simulink model "SMA_spring_pid"  (R2018a)
settings: Solver=ode15s  StartTime=0.0  StopTime=3.5  RelTol=1e-9  AbsTol=1e-9  EnableMultiTasking=on
values from neighbouring files (symbols this model uses):
  task_params = struct    [run.m]
undefined symbols (not defined in the file or in its folder): params_BIAS
settings Model: Creator=Gianluca  LastModifiedBy=tim
settings SolverCC: AutoScaleAbsTol=off
settings DataIOCC: LimitDataPoints=on  SaveFormat=Array
settings OptimizationCC: LifeSpan=inf
settings DebuggingCC: UnderspecifiedInitializationDetection=Classic  MergeDetectMultiDrivingBlocksExec=none  SolverPrmCheckMsg=warning  StateNameClashWarn=warning  SFUnexpectedBacktrackingDiag=warning  SFNoUnconditionalDefaultTransitionDiag=warning  SFExecutionAtInitializationDiag=none
settings HardwareCC: ProdBitPerPointer=32  ProdBitPerSizeT=32  ProdBitPerPtrDiffT=32  ProdLargestAtomicFloat=None  ProdIntDivRoundTo=Undefined  ProdEndianess=Unspecified  ProdWordSize=32  ProdHWDeviceType=32-bit Generic
settings ModelReferenceCC: PropagateSignalLabelsOutOfModel=off
settings CodeAppCC: StateflowObjectComments=on
settings GRTTargetCC: TargetLangStandard=C89/C90 (ANSI)  GeneratePreprocessorConditionals=Disable all
settings ConfigComp: CovMetricSettings=dw  CovHtmlReporting=on  CovSaveCumulativeToWorkspaceVar=on  CovSaveSingleToWorkspaceVar=on  CovExternalEMLEnable=off

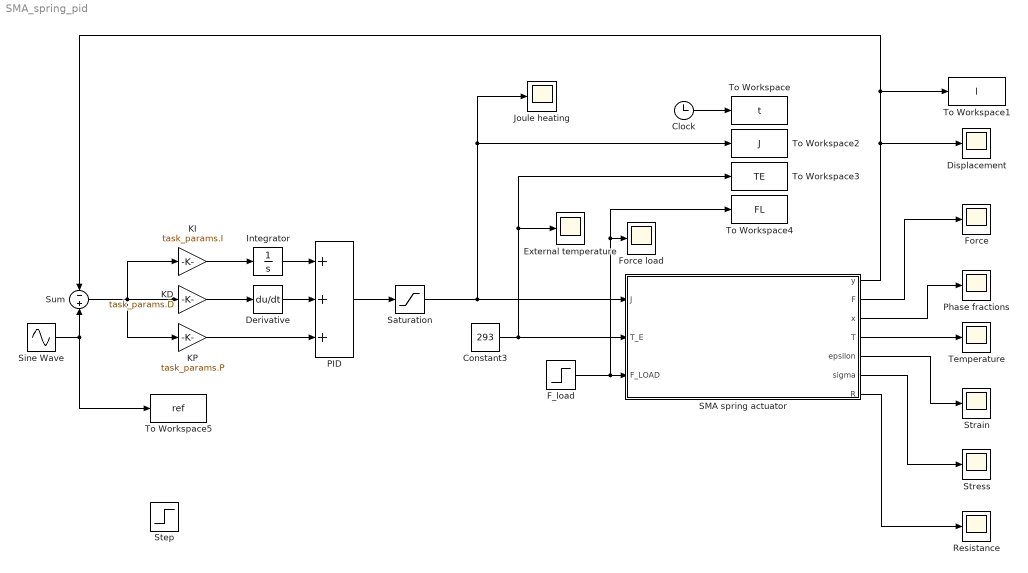
== system SMA_spring_pid ==
  " Force load" : Scope
  Clock : Clock
  Constant3 : Constant  Value=293
  Derivative : Derivative
  Displacement : Scope
  External temperature : Scope
  F_load : Step  After=0.05*0  SampleTime=0
  Force : Scope
  Integrator : Integrator
  Joule heating : Scope
  KD : Gain  Gain=task_params.D
  KI : Gain  Gain=task_params.I
  KP : Gain  Gain=task_params.P
  PID : Sum  Inputs=+++
  Phase fractions : Scope
  Resistance : Scope
  SMA spring actuator : Subsystem
      mask Display:
      | color('black');
      | patch(3*[-1 1 1 -1],1.1*[-1 -1 1 1],[1 1 1]);
      | patch([-1.6 -0.8],[-0.9 0.3],[0 0 0]);
      | patch([-0.8 1.2],[0.3 0.3],[0 0 0]);
      | patch([1.6 0.8],[0.9 -0.3],[0 0 0]);
      | patch([0.8 -1.2],[-0.3 -0.3],[0 0 0]);
      | disp('SMA spring');
      | 
      | color('blue');
      | port_label('input', 1, 'J [W]','texmode','on');
      | port_label('input', 2, 'T_E [K]','texmode','on');
      | port_label('input', 3, 'F_{LOAD} [N]','texmode','on');
      | 
      | color('red');
      | port_label('output', 1, 'y [m]','texmode','on');
      | port_label('output', 2, 'F [N]','texmode','on');
      | port_label('output', 3, 'x_+, x_-, x_A [-]','texmode','on');
      | port_label('output', 4, 'T [K]','texmode','on');
      | port_label('output', 5, '\epsilon [-]','texmode','on');
      | port_label('output', 6, '\sigma [Pa]','texmode','on');
      | port_label('output', 7, 'R [\Omega]','texmode','on');
  Saturation : Saturate  UpperLimit=0.25  LowerLimit=0  ZeroCross=off
  Sine Wave : Sin  Amplitude=task_params.sine_A  Bias=task_params.sine_bias  Frequency=2 * pi * task_params.sine_f  SampleTime=0
  Step : Step  Time=0  After=0.25*0.5  SampleTime=0
  Strain : Scope
  Stress : Scope
  Sum : Sum  Inputs=-+
  Temperature : Scope
  To Workspace : ToWorkspace  VariableName=t  SampleTime=0.01
  To Workspace1 : ToWorkspace  VariableName=l  SampleTime=0.01
  To Workspace2 : ToWorkspace  VariableName=J  SampleTime=0.01
  To Workspace3 : ToWorkspace  VariableName=TE  SampleTime=0.01
  To Workspace4 : ToWorkspace  VariableName=FL  SampleTime=0.01
  To Workspace5 : ToWorkspace  VariableName=ref  SampleTime=0.01
  wires:
  Constant3/1 -> To Workspace3/1, External temperature/1, SMA spring actuator/2(T_E)
  F_load/1 -> To Workspace4/1, " Force load"/1, SMA spring actuator/3(F_LOAD)
  SMA spring actuator/1(y) -> To Workspace1/1, Sum/1, Displacement/1
  SMA spring actuator/2(F) -> Force/1
  SMA spring actuator/3(x) -> Phase fractions/1
  SMA spring actuator/4(T) -> Temperature/1
  SMA spring actuator/5(epsilon) -> Strain/1
  SMA spring actuator/6(sigma) -> Stress/1
  SMA spring actuator/7(R) -> Resistance/1
  PID/1 -> Saturation/1
  Clock/1 -> To Workspace/1
  Saturation/1 -> Joule heating/1, To Workspace2/1, SMA spring actuator/1(J)
  Integrator/1 -> PID/1
  KP/1 -> PID/3
  Derivative/1 -> PID/2
  KI/1 -> Integrator/1
  Sum/1 -> KP/1, KI/1, KD/1
  KD/1 -> Derivative/1
  Sine Wave/1 -> To Workspace5/1, Sum/2

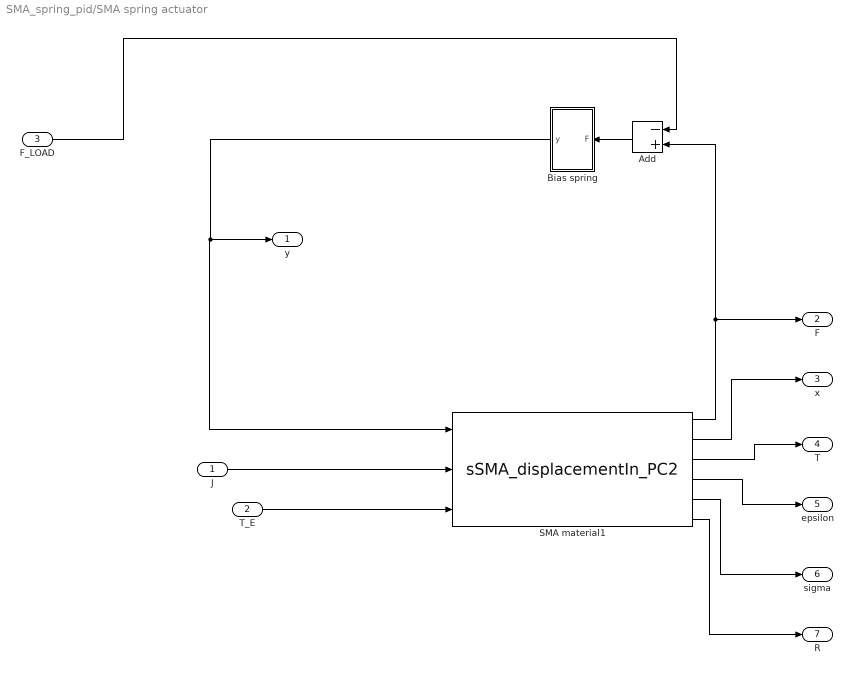
== system SMA_spring_pid/SMA spring actuator ==
  J : Inport
  T_E : Inport  Port=2
  F_LOAD : Inport  Port=3
  Add : Sum  Inputs=-+
  Bias spring : Subsystem
  SMA material1 : M-S-Function  FunctionName=sSMA_displacementIn_PC2  Parameters=params_PC2, initConds_PC2
      mask Display:
      | color('black');
      | patch(3*[-1 1 1 -1],1.1*[-1 -1 1 1],[1 1 1]);
      | patch([-1.6 -0.8],[-0.9 0.3],[0 0 0]);
      | patch([-0.8 1.2],[0.3 0.3],[0 0 0]);
      | patch([1.6 0.8],[0.9 -0.3],[0 0 0]);
      | patch([0.8 -1.2],[-0.3 -0.3],[0 0 0]);
      | disp('SMA');
      | 
      | color('blue');
      | port_label('input', 1, 'y [m]','texmode','on');
      | port_label('input', 2, 'J [W]','texmode','on');
      | port_label('input', 3, 'T_E [K]','texmode','on');
      | 
      | color('red');
      | port_label('output', 1, 'F [N]','texmode','on');
      | port_label('output', 2, 'x_+, x_-, x_A [-]','texmode','on');
      | port_label('output', 3, 'T [K]','texmode','on');
      | port_label('output', 4, '\epsilon [-]','texmode','on');
      | port_label('output', 5, '\sigma [Pa]','texmode','on');
      | port_label('output', 6, 'R [\Omega]','texmode','on');
  y : Outport
  F : Outport  Port=2
  x : Outport  Port=3
  T : Outport  Port=4
  epsilon : Outport  Port=5
  sigma : Outport  Port=6
  R : Outport  Port=7
  wires:
  J/1 -> SMA material1/2
  T_E/1 -> SMA material1/3
  F_LOAD/1 -> Add/1
  Add/1 -> Bias spring/1(F)
  SMA material1/5 -> sigma/1
  SMA material1/1 -> F/1, Add/2
  SMA material1/2 -> x/1
  SMA material1/3 -> T/1
  SMA material1/4 -> epsilon/1
  SMA material1/6 -> R/1
  Bias spring/1(y) -> y/1, SMA material1/1

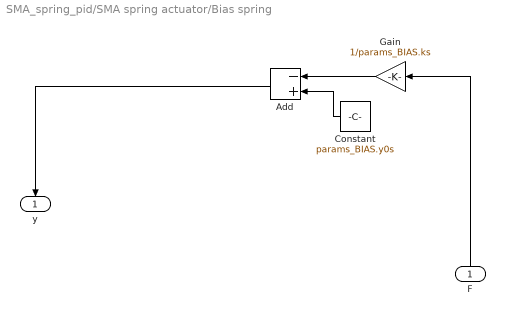
== system SMA_spring_pid/SMA spring actuator/Bias spring ==
  F : Inport
  Add : Sum  Inputs=-+
  Constant : Constant  Value=params_BIAS.y0s
  Gain : Gain  Gain=1/params_BIAS.ks
  y : Outport
  wires:
  Add/1 -> y/1
  F/1 -> Gain/1
  Constant/1 -> Add/2
  Gain/1 -> Add/1
